simulink model "TClabControlSat_R2016a"  (R2016a)
settings: Solver=VariableStepAuto  SolverMode=SingleTasking  StartTime=0.0  StopTime=600  RelTol=1e-3
StartFcn:
  | reset_temp
values from neighbouring files (symbols this model uses):
  Dref = ref-yroom    (= 7)    [setupModelParametersDT.m]    (also in setupModelParametersSat.m = 37)
  ki = 0.1    [setupModelParametersDT.m]    (also in setupModelParametersSat.m)
  kp = 8.75    [setupModelParametersDT.m]    (also in setupModelParametersSat.m)
  P = tf([-tau/2, 1],[tau/2 1])*tf(K,[1 a])    [setupModelParametersDT.m]    (also in setupModelParametersSat.m)
  yroom = 23    [setupModelParametersDT.m]    (also in setupModelParametersSat.m)
settings Model: Creator=jamess  LastModifiedBy=jamessaunderson
settings DebuggingCC: SFUnexpectedBacktrackingDiag=error  SFNoUnconditionalDefaultTransitionDiag=error
settings GRTTargetCC: TargetLangStandard=C99 (ISO)
settings ConfigComp: CovMetricSettings=dwe  CovHtmlReporting=off  CovSaveCumulativeToWorkspaceVar=off  CovSaveSingleToWorkspaceVar=off  CovExternalEMLEnable=on

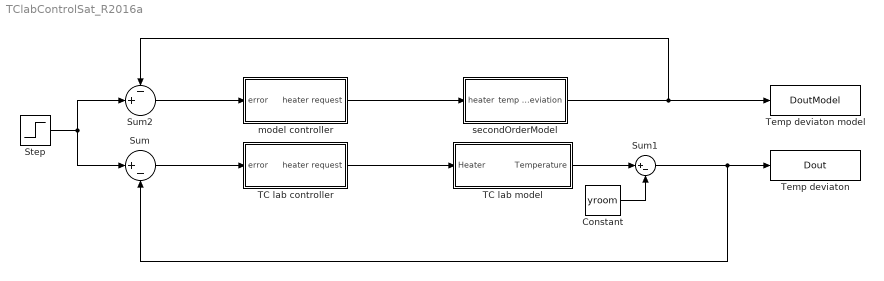
== system TClabControlSat_R2016a ==
  Constant : Constant  Value=yroom
  Step : Step  Time=0  After=Dref  SampleTime=0
  Sum : Sum  Inputs=|+-
  Sum1 : Sum  Inputs=|+-
  Sum2 : Sum  Inputs=-+|
  TC lab controller : Subsystem
  TC lab model : Subsystem
  Temp deviaton : ToWorkspace  VariableName=Dout  SaveFormat=Timeseries  SampleTime=-1
  Temp deviaton model : ToWorkspace  VariableName=DoutModel  SaveFormat=Timeseries  SampleTime=-1
  "model controller " : Subsystem
  secondOrderModel : Subsystem
  wires:
  secondOrderModel/1(temp deviation) -> Temp deviaton model/1, Sum2/1
  TC lab controller/1(heater request) -> TC lab model/1(Heater)
  Step/1 -> Sum/1, Sum2/2
  Sum1/1 -> Temp deviaton/1, Sum/2
  TC lab model/1(Temperature) -> Sum1/1
  Constant/1 -> Sum1/2
  "model controller "/1(heater request) -> secondOrderModel/1(heater)
  Sum/1 -> TC lab controller/1(error)
  Sum2/1 -> "model controller "/1(error)

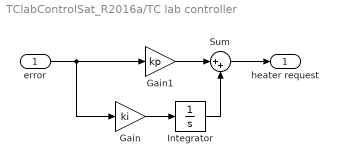
== system TClabControlSat_R2016a/TC lab controller ==
  error : Inport
  Gain : Gain  Gain=ki
  Gain1 : Gain  Gain=kp
  Integrator : Integrator
  Sum : Sum  Inputs=|++
  heater request : Outport
  wires:
  error/1 -> Gain/1, Gain1/1
  Sum/1 -> heater request/1
  Gain/1 -> Integrator/1
  Gain1/1 -> Sum/1
  Integrator/1 -> Sum/2

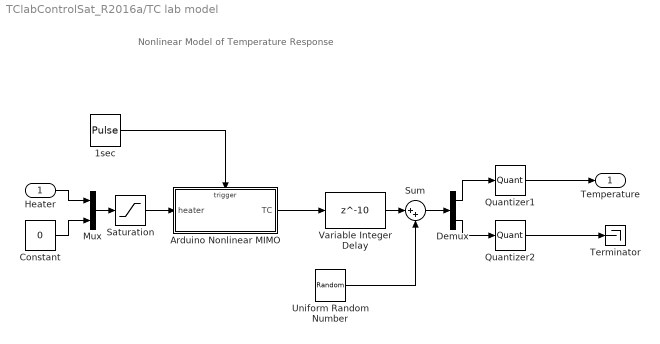
== system TClabControlSat_R2016a/TC lab model ==
  note: Nonlinear Model of Temperature Response
  Heater : Inport
  1sec : DiscretePulseGenerator  PulseType=Time based  Period=1  PulseWidth=50
  Arduino Nonlinear MIMO : Subsystem  TreatAsAtomicUnit=on
  Constant : Constant  Value=0
  Demux : Demux  Outputs=2
  Mux : Mux  Inputs=2
  Quantizer1 : Quantizer
  Quantizer2 : Quantizer
  Saturation : Saturate  UpperLimit=100  LowerLimit=0
  Sum : Sum  Inputs=|++
  Terminator : Terminator
  Uniform Random Number : UniformRandomNumber  Minimum=[-1;-1]  Maximum=[1;1]  SampleTime=1
  Variable Integer Delay : Delay  DelayLength=10  InitialCondition=23  SampleTime=1
  Temperature : Outport
  wires:
  1sec/1 -> Arduino Nonlinear MIMO/Trigger
  Constant/1 -> Mux/2
  Heater/1 -> Mux/1
  Demux/1 -> Quantizer1/1
  Demux/2 -> Quantizer2/1
  Quantizer1/1 -> Temperature/1
  Quantizer2/1 -> Terminator/1
  Arduino Nonlinear MIMO/1(TC) -> Variable Integer Delay/1
  Uniform Random Number/1 -> Sum/2
  Sum/1 -> Demux/1
  Variable Integer Delay/1 -> Sum/1
  Mux/1 -> Saturation/1
  Saturation/1 -> Arduino Nonlinear MIMO/1(heater)

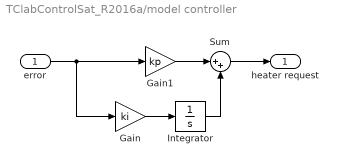
== system TClabControlSat_R2016a/model controller  ==
  error : Inport
  Gain : Gain  Gain=ki
  Gain1 : Gain  Gain=kp
  Integrator : Integrator
  Sum : Sum  Inputs=|++
  heater request : Outport
  wires:
  error/1 -> Gain/1, Gain1/1
  Sum/1 -> heater request/1
  Gain/1 -> Integrator/1
  Gain1/1 -> Sum/1
  Integrator/1 -> Sum/2

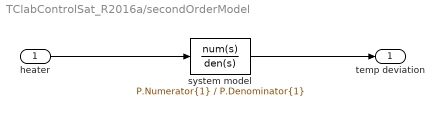
== system TClabControlSat_R2016a/secondOrderModel ==
  heater : Inport
  system model : TransferFcn  Numerator=P.Numerator{1}  Denominator=P.Denominator{1}
  temp deviation : Outport
  wires:
  heater/1 -> system model/1
  system model/1 -> temp deviation/1

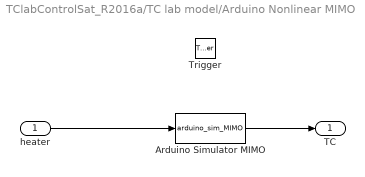
== system TClabControlSat_R2016a/TC lab model/Arduino Nonlinear MIMO ==
  heater : Inport
  Trigger : TriggerPort  VariantControl=Variant
  Arduino Simulator MIMO : MATLABFcn  MATLABFcn=arduino_sim_MIMO
  TC : Outport  InitialOutput=23
  wires:
  Arduino Simulator MIMO/1 -> TC/1
  heater/1 -> Arduino Simulator MIMO/1
